simulink model "stabilizacja_lqr"  (R2013b)
settings: Solver=ode4  StartTime=0.0  StopTime=tSim  FixedStep=h  RelTol=1e-3
values from neighbouring files (symbols this model uses):
  K = [-6.6845,-51.6047,-9.6527,-10]    [launcher_simulink.m]    (also in strojenie_lqr.m = lqr(A,B,Q,R); strojenie_pid_pozycja.m = 1 / (M * s^2 + b * s); strojenie_silnik.m = 0.0274)
  modelSelect = 'full'    [launcher_script.m]    (also in launcher_simulink.m = 'linear')
  N = K(4)    [launcher_simulink.m]
  params = [M,m,L,I,b,g]    [launcher_script.m]    (also in launcher_simulink.m)
  state0 = [thetaDot0;theta0;xDot0;x0]    [launcher_script.m]    (also in launcher_simulink.m; sFunction.m = [])
settings Model: Creator=JAR  LastModifiedBy=JAR

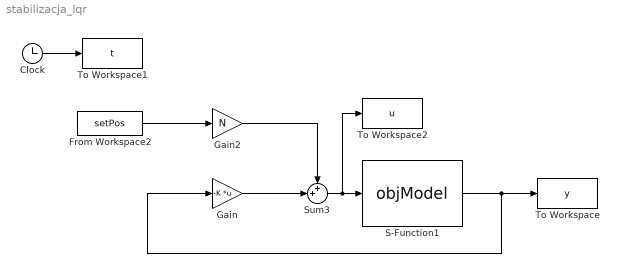
== system stabilizacja_lqr ==
  Clock : Clock
  From Workspace2 : FromWorkspace  VariableName=setPos  SampleTime=0
  Gain : Gain  Gain=-K  Multiplication=Matrix(K*u)
  Gain2 : Gain  Gain=N
  S-Function1 : S-Function  FunctionName=objModel  Parameters=state0,params,modelSelect  EnableBusSupport=off
  Sum3 : Sum  Inputs=++|
  To Workspace : ToWorkspace  VariableName=y  SampleTime=-1
  To Workspace1 : ToWorkspace  VariableName=t  SampleTime=-1
  To Workspace2 : ToWorkspace  VariableName=u  SampleTime=-1
  wires:
  Clock/1 -> To Workspace1/1
  From Workspace2/1 -> Gain2/1
  Sum3/1 -> To Workspace2/1, S-Function1/1
  Gain2/1 -> Sum3/1
  Gain/1 -> Sum3/2
  S-Function1/1 -> Gain/1, To Workspace/1
